simulink model "ex3_sim1m"  (R2022b)
settings: Solver=ode45  StartTime=0.0  StopTime=2  MaxStep=0.0001  RelTol=1e-3
undefined symbols (not defined in the file): bit, d, denC, denH, denPc, denQ, denQP, mot, numC, numH, numPc, numQ, numQP, pulse2deg, r, rads2rpm, rpm2rads, Ts, umax
settings Model: Creator=loren  LastModifiedBy=loren
settings DataIOCC: ReturnWorkspaceOutputs=off

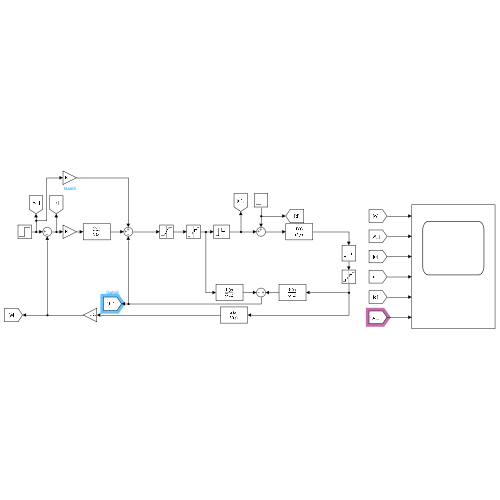
[thumbnail: Simulink's stored preview of the top-level diagram]
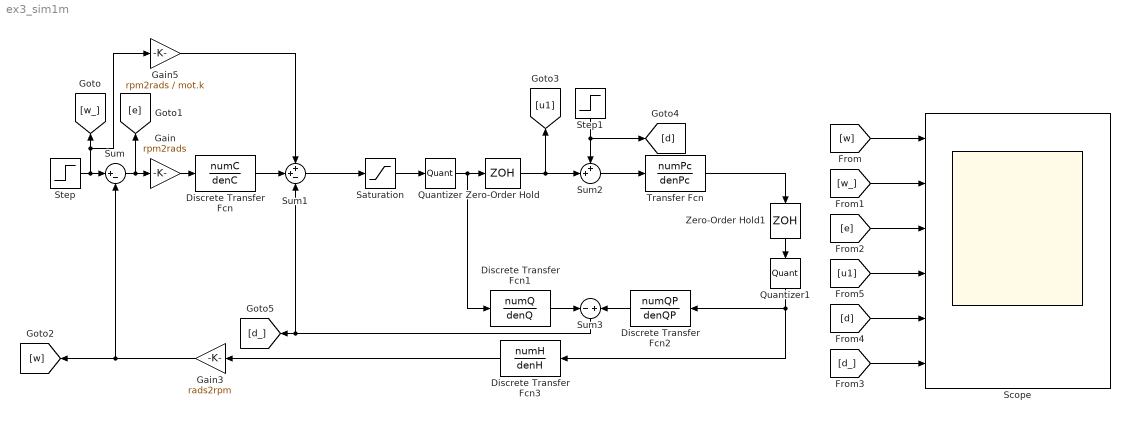
== system ex3_sim1m ==
  Discrete Transfer Fcn : DiscreteTransferFcn  Numerator=numC  Denominator=denC  SampleTime=Ts
  Discrete Transfer Fcn1 : DiscreteTransferFcn  Numerator=numQ  Denominator=denQ  SampleTime=Ts
  Discrete Transfer Fcn2 : DiscreteTransferFcn  Numerator=numQP  Denominator=denQP  SampleTime=Ts
  Discrete Transfer Fcn3 : DiscreteTransferFcn  Numerator=numH  Denominator=denH  SampleTime=Ts
  Gain : Gain  Gain=rpm2rads
  Gain3 : Gain  Gain=rads2rpm
  Gain5 : Gain  Gain=rpm2rads / mot.k
  Quantizer : Quantizer  QuantizationInterval=2 * umax / 2^bit
  Quantizer1 : Quantizer  QuantizationInterval=pulse2deg * deg2rad
  Saturation : Saturate  UpperLimit=umax  LowerLimit=-umax
  Scope : Scope  NumInputPorts=6
  Step : Step  Time=r.t  After=r.A  SampleTime=0
  Step1 : Step  Time=d.t  After=d.A  SampleTime=0
  Sum : Sum  Inputs=|+-
  Sum1 : Sum  Inputs=++-
  Sum2 : Sum  Inputs=++|
  Sum3 : Sum  Inputs=-|+
  Transfer Fcn : TransferFcn  Numerator=numPc  Denominator=denPc
  Zero-Order Hold : ZeroOrderHold  SampleTime=Ts
  Zero-Order Hold1 : ZeroOrderHold  SampleTime=Ts
  wires:
  Step/1 -> Gain5/1, [w_], Sum/1
  Sum/1 -> [e], Gain/1
  Sum1/1 -> Saturation/1
  Saturation/1 -> Quantizer/1
  Quantizer/1 -> Discrete Transfer Fcn1/1, Zero-Order Hold/1
  Zero-Order Hold/1 -> Sum2/2, [u1]
  Sum2/1 -> Transfer Fcn/1
  Zero-Order Hold1/1 -> Quantizer1/1
  Discrete Transfer Fcn2/1 -> Sum3/2
  Discrete Transfer Fcn1/1 -> Sum3/1
  Sum3/1 -> Sum1/3, [d_]
  Discrete Transfer Fcn3/1 -> Gain3/1
  Step1/1 -> Sum2/1, [d]
  Gain/1 -> Discrete Transfer Fcn/1
  Quantizer1/1 -> Discrete Transfer Fcn3/1, Discrete Transfer Fcn2/1
  Gain3/1 -> [w], Sum/2
  [w] -> Scope/1
  [w_] -> Scope/2
  [e] -> Scope/3
  [u1] -> Scope/4
  [d] -> Scope/5
  [d_] -> Scope/6
  Transfer Fcn/1 -> Zero-Order Hold1/1
  Discrete Transfer Fcn/1 -> Sum1/2
  Gain5/1 -> Sum1/1
